simulink model "fluid_animated_restored_from_autosave"  (R2018b)
settings: Solver=ode45  StartTime=0.0  StopTime=50.0  MaxStep=0.01  RelTol=1e-3  EnableMultiTasking=on
undefined symbols (not defined in the file or in its folder): A, animate_fluid_tank, B, C, D, g, omega_0, rho, Xo
settings Model: Creator=buddyugwumba1  LastModifiedBy=buddyugwumba1
settings DataIOCC: LimitDataPoints=on  SaveFormat=Array  SignalLoggingSaveFormat=ModelDataLogs
settings OptimizationCC: InitFltsAndDblsToZero=on  LifeSpan=inf
settings DebuggingCC: SaveWithParameterizedLinksMsg=none  UnderspecifiedInitializationDetection=Classic  MergeDetectMultiDrivingBlocksExec=none  SignalResolutionControl=TryResolveAllWithWarning  SolverPrmCheckMsg=warning  MultiTaskDSMMsg=warning  MultiTaskCondExecSysMsg=none  SFUnexpectedBacktrackingDiag=warning  SFNoUnconditionalDefaultTransitionDiag=warning  SFExecutionAtInitializationDiag=none
settings HardwareCC: ProdBitPerPointer=32  ProdBitPerSizeT=32  ProdBitPerPtrDiffT=32  ProdLargestAtomicFloat=None  ProdIntDivRoundTo=Undefined  ProdEndianess=Unspecified  ProdWordSize=32  ProdHWDeviceType=32-bit Generic
settings ModelReferenceCC: PropagateSignalLabelsOutOfModel=off
settings CodeAppCC: StateflowObjectComments=on
settings GRTTargetCC: TargetFcnLib=ansi_tfl_tmw.mat  TargetLangStandard=C89/C90 (ANSI)  CombineOutputUpdateFcns=off  GRTInterface=on
settings ConfigComp: CovMetricSettings=dw  CovHtmlReporting=on  CovSaveCumulativeToWorkspaceVar=on  CovSaveSingleToWorkspaceVar=on

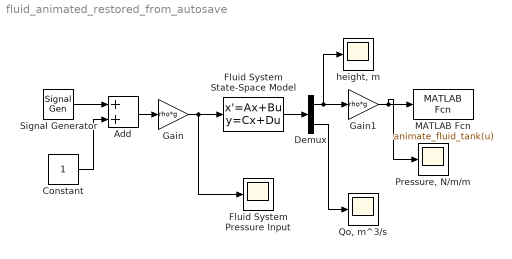
== system fluid_animated_restored_from_autosave ==
  Add : Sum
  Constant : Constant
  Demux : Demux  Outputs=[3,1]
  Fluid System Pressure Input : Scope
  Fluid System State-Space Model : StateSpace  A=A  B=B  C=C  D=D  InitialCondition=Xo
  Gain : Gain  Gain=rho*g
  Gain1 : Gain  Gain=rho*g
  MATLAB Fcn : MATLABFcn  MATLABFcn=animate_fluid_tank(u)  SampleTime=0.01
  "Pressure, N/m/m" : Scope
  "Qo, m^3/s" : Scope
  Signal Generator : SignalGenerator  Frequency=omega_0  Units=rad/sec
  "height, m" : Scope
  wires:
  Add/1 -> Gain/1
  Constant/1 -> Add/2
  Signal Generator/1 -> Add/1
  Fluid System State-Space Model/1 -> Demux/1
  Demux/1 -> "height, m"/1, Gain1/1
  Demux/2 -> "Qo, m^3/s"/1
  Gain/1 -> Fluid System State-Space Model/1, Fluid System Pressure Input/1
  Gain1/1 -> MATLAB Fcn/1, "Pressure, N/m/m"/1
